simulink model "cstd2_sim_lqg"  (R2012b)
settings: Solver=ode45  StartTime=0.0  StopTime=15  FixedStep=0.005  RelTol=1e-3
values from neighbouring files (symbols this model uses):
  A_obsv = A    [cstd2_design.m]
  B_obsv = B    [cstd2_design.m]
  C_obsv = C    [cstd2_design.m]
  D_obsv = D    [cstd2_design.m]
  F = -lqr(A, B, Q_lqr, R_lqr)    [cstd2_design.m]
  sys = ss1    [cstd2_design.m]
  V = 0.1*(360/293.99)    (= 0.122453144665)    [cstd2_design.m]
undefined symbols (not defined in the file or in its folder): sigbuilder_block
settings Model: ExtModeTrigDuration=30000  Creator=maglev  LastModifiedBy=Michael
settings DataIOCC: LimitDataPoints=off  MaxDataPoints=5000000  SaveFormat=StructureWithTime  SignalLoggingSaveFormat=ModelDataLogs  SaveOutput=off  SignalLogging=off  SaveTime=off
settings DebuggingCC: MultiTaskDSMMsg=warning  MultiTaskCondExecSysMsg=none  FcnCallInpInsideContextMsg=UseLocalSettings  StrictBusMsg=None
settings HardwareCC: ProdIntDivRoundTo=Zero  ProdEndianess=LittleEndian  ProdHWDeviceType=Generic->32-bit x86 compatible
settings RTWCC: SystemTargetFile=rtwin.tlc  TemplateMakefile=rtwin.tmf  Description=Real-Time Windows Target  ProcessScript=rtwin_make_rtw_hook  IncludeERTFirstTime=on
settings CodeAppCC: MaxIdLength=95  CustomSymbolStrType=$N$R$M_T  InternalIdentifier=Shortened
settings RTWinTargetCC: TargetLibSuffix=_rtwin.lib  TargetPreCompLibLocation=C:\Program Files\MATLAB\R2012b\toolbox\rtw\targets\rtwin\lib\win64  RTWinDir=C:/PROGRA~1/MATLAB/R2012b/toolbox/rtw/targets/rtwin  TargetArch=win64

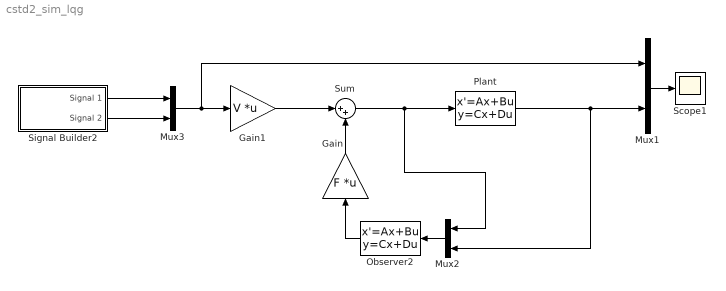
== system cstd2_sim_lqg ==
  Gain : Gain  Gain=F  Multiplication=Matrix(K*u)
  Gain1 : Gain  Gain=V  Multiplication=Matrix(K*u)
  Mux1 : Mux  Inputs=2
  Mux2 : Mux  Inputs=2
  Mux3 : Mux  Inputs=2
  Observer2 : StateSpace  A=A_obsv  B=B_obsv  C=C_obsv  D=D_obsv
  Plant : StateSpace  A=sys.A  B=sys.B  C=sys.C  D=sys.D  X0=[0, 0, 0, 0]
  Scope1 : Scope
      settings: SaveName=data
  Signal Builder2 : Subsystem  Tag=STV Subsys  LoadFcn=sigbuilder_block('load');  StartFcn=sigbuilder_block('start');  StopFcn=sigbuilder_block('stop');  ClipboardFcn=sigbuilder_block('clipboard');  mask(Sigbuilder block){}
      mask help: Simulink:masks:SigbuilderBlock_MD
      mask init:
      | if ~strcmp(get_param(bdroot(gcbh),'SimulationStatus'),'stopped') tuvar = sigbuilder_block('maskInit'); end
      settings: CopyFcn=sigbuilder_block('copy');  DeleteFcn=sigbuilder_block('delete');  ModelCloseFcn=sigbuilder_block('modelClose');  PreSaveFcn=sigbuilder_block('preSave');  PauseFcn=sigbuilder_block('pause');  ContinueFcn=sigbuilder_block('continue');  NameChangeFcn=sigbuilder_block('namechange');  OpenFcn=sigbuilder_block('open',[437.25 199.5 550.5 399.75 ]);  CloseFcn=sigbuilder_block('close');
      mask Display: plot(0, 0, 100, 100,[2, 2, 32, 32, 2], [68, 8, 8, 68, 68],[32, 2], [38, 38], [32, 19, 2],[53, 60, 44], [32, 17, 17, 2],[16, 16, 31, 31]);txt = getActiveGroup(gcbh);text(2, 100, txt,'verticalAlignment', 'top');
  Sum : Sum  Inputs=|++
  wires:
  Mux2/1 -> Observer2/1
  Mux3/1 -> Mux1/1, Gain1/1
  Plant/1 -> Mux2/2, Mux1/2
  Observer2/1 -> Gain/1
  Gain/1 -> Sum/2
  Sum/1 -> Plant/1, Mux2/1
  Gain1/1 -> Sum/1
  Mux1/1 -> Scope1/1
  Signal Builder2/1(Signal 1) -> Mux3/1
  Signal Builder2/2(Signal 2) -> Mux3/2

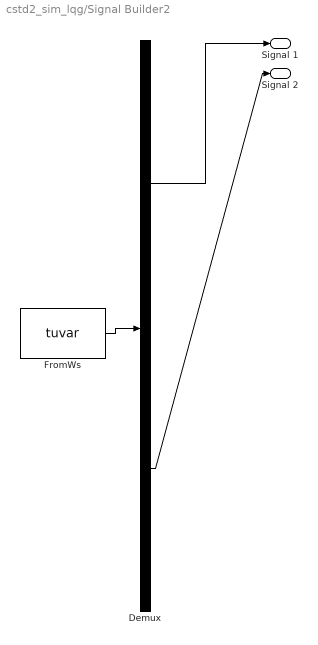
== system cstd2_sim_lqg/Signal Builder2 ==
  Demux : Demux  Tag=STV Demux  Outputs=2
  FromWs : FromWorkspace  Tag=STV FromWs  VariableName=tuvar  SampleTime=0
      SigBuilderData=|
      | common.afterFinalStr = 'Extrapolate'
      | common.sampleTime = 0
      | dataSet.timeRange = [0 15]
      | dataSet.name = 'Group 1'
      | sbobj.Groups.Name = 'Group 1'
      | sbobj.Groups.Signals(1).Name = 'Signal 1'
      | sbobj.Groups.Signals(1).XData = [0 5 5 6 6 7 7 8 8 9 9 10 10 11 11 12 12 15]
      | sbobj.Groups.Signals(1).YData = [0 0 1 1 -0.01 0 -1 -1 0 0 1 1 0 0 -1 -1 0 0]
      | sbobj.Groups.Signals(2).Name = 'Signal 2'
      | sbobj.Groups.Signals(2).XData = [0 2.5 3.5 3.5 4.5 5.5 5.5 6.5 6.5 7.5 7.5 8.5 8.5 9.5 9.5 10.5 10.5 11.5 11.5 12.5 12.5 15]
      | sbobj.Groups.Signals(2).YData = [0 0 -0.5 0.5 0 0 0.5 0.5 0 0 -0.5 -0.5 0 0 -0.5 -0.5 0 0 0.5 0.5 0 0]
      | sbobj.Groups.TimeRange = [0 15]
  Signal 1 : Outport  Tag=STV Outport
  Signal 2 : Outport  Tag=STV Outport  Port=2
  wires:
  FromWs/1 -> Demux/1
  Demux/1 -> Signal 1/1
  Demux/2 -> Signal 2/1
